simulink model "img_Closedloop"  (R2015b)
settings: Solver=VariableStepAuto  StartTime=0.0  StopTime=600  RelTol=1e-3
values from neighbouring files (symbols this model uses):
  Cp = xlsread(filename)    [Cpfun.m]
undefined symbols (not defined in the file or in its folder): A1, a11, a12, a13, A2, a21, a22, a23, A3, a31, a32, a33, A4, A5, b11, b12, b21, b22, b31, b32, beta_opt, Cr, eta, Jr, lambda, lambda_opt, phi, R, Rho, vf
settings Model: Creator=alino  LastModifiedBy=alino

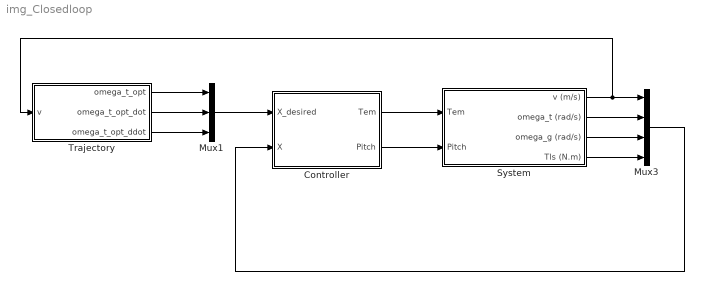
== system img_Closedloop ==
  Controller : Subsystem
  Mux1 : Mux  Inputs=3
  Mux3 : Mux
  System : Subsystem
  Trajectory : Subsystem
  wires:
  Mux3/1 -> Controller/2(X)
  Mux1/1 -> Controller/1(X_desired)
  Trajectory/2(omega_t_opt_dot) -> Mux1/2
  Trajectory/1(omega_t_opt) -> Mux1/1
  Controller/1(Tem) -> System/1(Tem)
  Controller/2(Pitch) -> System/2(Pitch)
  System/3(omega_g (rad/s)) -> Mux3/3
  System/4(Tls (N.m)) -> Mux3/4
  System/2(omega_t (rad/s)) -> Mux3/2
  System/1(v (m/s)) -> Trajectory/1(v), Mux3/1
  Trajectory/3(omega_t_opt_ddot) -> Mux1/3

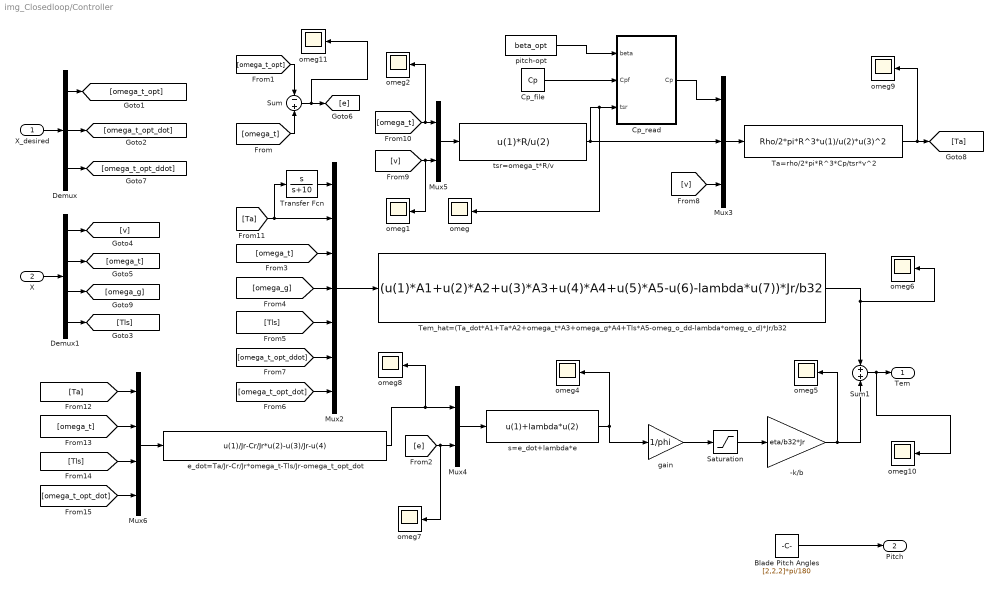
== system img_Closedloop/Controller ==
  X_desired : Inport
  X : Inport  Port=2
  -k/b : Gain  Gain=eta/b32*Jr
  Blade Pitch Angles : Constant  Value=[2,2,2]*pi/180
  Cp_file : Constant  Value=Cp
  Cp_read : MATLAB Function  TreatAsAtomicUnit=on
  Demux : Demux  Outputs=3
  Demux1 : Demux
  Mux2 : Mux  Inputs=7
  Mux3 : Mux  Inputs=3
  Mux4 : Mux  Inputs=2
  Mux5 : Mux  Inputs=2
  Mux6 : Mux
  Saturation : Saturate  UpperLimit=1  LowerLimit=-1
  Sum : Sum  Inputs=-+
  Sum1 : Sum  Inputs=+|+
  Ta=rho/2*pi*R^3*Cp/tsr*v^2 : Fcn  Expr=Rho/2*pi*R^3*u(1)/u(2)*u(3)^2
  Tem_hat=(Ta_dot*A1+Ta*A2+omega_t*A3+omega_g*A4+Tls*A5-omeg_o_dd-lambda*omeg_o_d)*Jr/b32 : Fcn  Expr=(u(1)*A1+u(2)*A2+u(3)*A3+u(4)*A4+u(5)*A5-u(6)-lambda*u(7))*Jr/b32
  Transfer Fcn : TransferFcn  Numerator=[1 0]  Denominator=[1 10]
  e_dot=Ta/Jr-Cr/Jr*omega_t-Tls/Jr-omega_t_opt_dot : Fcn  Expr=u(1)/Jr-Cr/Jr*u(2)-u(3)/Jr-u(4)
  gain : Gain  Gain=1/phi
  omeg{,1..2,4..11} (11 alike) : Scope
  pitch-opt : Constant  Value=beta_opt
  s=e_dot+lambda*e : Fcn  Expr=u(1)+lambda*u(2)
  tsr=omega_t*R/v : Fcn  Expr=u(1)*R/u(2)
  Tem : Outport
  Pitch : Outport  Port=2
  wires:
  X_desired/1 -> Demux/1
  X/1 -> Demux1/1
  Tem_hat=(Ta_dot*A1+Ta*A2+omega_t*A3+omega_g*A4+Tls*A5-omeg_o_dd-lambda*omeg_o_d)*Jr/b32/1 -> Sum1/1, omeg6/1
  -k/b/1 -> Sum1/2, omeg5/1
  Mux2/1 -> Tem_hat=(Ta_dot*A1+Ta*A2+omega_t*A3+omega_g*A4+Tls*A5-omeg_o_dd-lambda*omeg_o_d)*Jr/b32/1
  Mux4/1 -> s=e_dot+lambda*e/1
  [omega_t] -> Mux2/3
  Demux/1 -> [omega_t_opt]
  Demux/2 -> [omega_t_opt_dot]
  Demux1/1 -> [v]
  Demux1/2 -> [omega_t]
  Demux1/3 -> [omega_g]
  Blade Pitch Angles/1 -> Pitch/1
  Demux1/4 -> [Tls]
  Sum/1 -> omeg11/1, [e]
  [omega_t] -> Sum/2
  [omega_t_opt] -> Sum/1
  [e] -> omeg7/1, Mux4/2
  Demux/3 -> [omega_t_opt_ddot]
  [omega_g] -> Mux2/4
  [Tls] -> Mux2/5
  Mux3/1 -> Ta=rho/2*pi*R^3*Cp/tsr*v^2/1
  [v] -> Mux3/3
  Mux5/1 -> tsr=omega_t*R/v/1
  [v] -> omeg1/1, Mux5/2
  [omega_t] -> omeg2/1, Mux5/1
  tsr=omega_t*R/v/1 -> Mux3/2, omeg/1, Cp_read/3(tsr)
  Ta=rho/2*pi*R^3*Cp/tsr*v^2/1 -> omeg9/1, [Ta]
  [Ta] -> Transfer Fcn/1, Mux2/2
  Transfer Fcn/1 -> Mux2/1
  Mux6/1 -> e_dot=Ta/Jr-Cr/Jr*omega_t-Tls/Jr-omega_t_opt_dot/1
  e_dot=Ta/Jr-Cr/Jr*omega_t-Tls/Jr-omega_t_opt_dot/1 -> omeg8/1, Mux4/1
  [Ta] -> Mux6/1
  [omega_t] -> Mux6/2
  [Tls] -> Mux6/3
  [omega_t_opt_dot] -> Mux6/4
  Cp_read/1(Cp) -> Mux3/1
  Cp_file/1 -> Cp_read/2(Cpf)
  pitch-opt/1 -> Cp_read/1(beta)
  Sum1/1 -> omeg10/1, Tem/1
  [omega_t_opt_dot] -> Mux2/7
  [omega_t_opt_ddot] -> Mux2/6
  s=e_dot+lambda*e/1 -> gain/1, omeg4/1
  Saturation/1 -> -k/b/1
  gain/1 -> Saturation/1

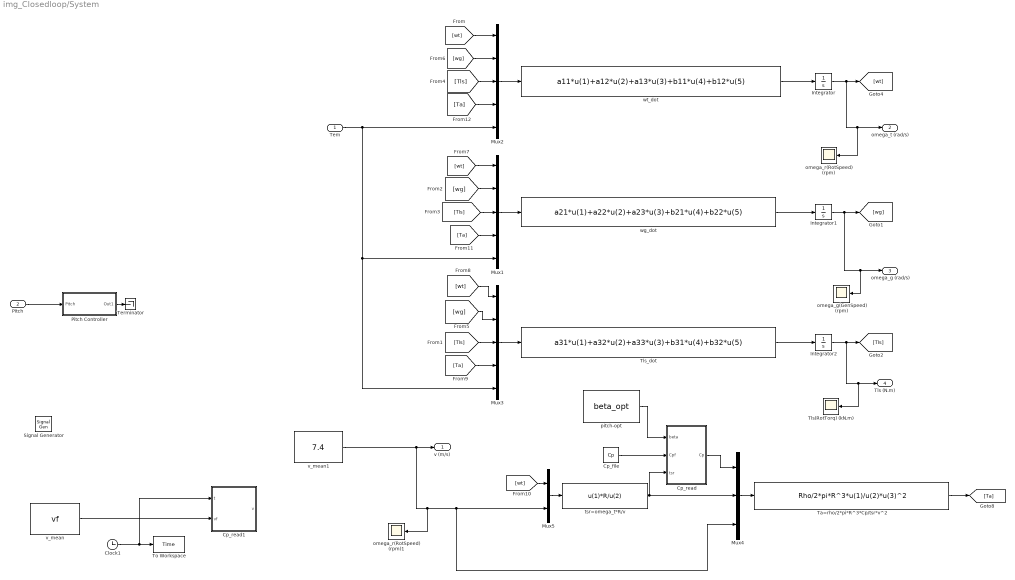
== system img_Closedloop/System ==
  Tem : Inport
  Pitch : Inport  Port=2
  Clock1 : Clock
  Cp_file : Constant  Value=Cp
  Cp_read : MATLAB Function  TreatAsAtomicUnit=on
  Cp_read1 : MATLAB Function  TreatAsAtomicUnit=on
  Integrator : Integrator  InitialCondition=2
  Integrator1 : Integrator  InitialCondition=2
  Integrator2 : Integrator
  Mux1 : Mux  Inputs=5
  Mux2 : Mux  Inputs=5
  Mux3 : Mux  Inputs=5
  Mux4 : Mux  Inputs=3
  Mux5 : Mux  Inputs=2
  Pitch Controller : Subsystem
  Signal Generator : SignalGenerator  WaveForm=random  Units=rad/sec
  Ta=rho/2*pi*R^3*Cp/tsr*v^2 : Fcn  Expr=Rho/2*pi*R^3*u(1)/u(2)*u(3)^2
  Terminator : Terminator
  Tls(RotTorq) (kN.m) : Scope
  Tls_dot : Fcn  Expr=a31*u(1)+a32*u(2)+a33*u(3)+b31*u(4)+b32*u(5)
  To Workspace : ToWorkspace  VariableName=Time  SampleTime=-1
  omega_g(GenSpeed) (rpm) : Scope
  omega_r(RotSpeed) (rpm) : Scope
  omega_r(RotSpeed) (rpm)1 : Scope
  pitch-opt : Constant  Value=beta_opt
  tsr=omega_t*R/v : Fcn  Expr=u(1)*R/u(2)
  v_mean : Constant  Value=vf
  v_mean1 : Constant  Value=7.4
  wg_dot : Fcn  Expr=a21*u(1)+a22*u(2)+a23*u(3)+b21*u(4)+b22*u(5)
  wt_dot : Fcn  Expr=a11*u(1)+a12*u(2)+a13*u(3)+b11*u(4)+b12*u(5)
  v (m/s) : Outport
  omega_t (rad/s) : Outport  Port=2
  omega_g (rad/s) : Outport  Port=3
  Tls (N.m) : Outport  Port=4
  wires:
  Clock1/1 -> Cp_read1/1(t), To Workspace/1
  Integrator/1 -> omega_t (rad/s)/1, omega_r(RotSpeed) (rpm)/1, [wt]
  Integrator1/1 -> omega_g(GenSpeed) (rpm)/1, omega_g (rad/s)/1, [wg]
  Integrator2/1 -> Tls(RotTorq) (kN.m)/1, Tls (N.m)/1, [Tls]
  Pitch/1 -> Pitch Controller/1(Pitch)
  Mux2/1 -> wt_dot/1
  Mux1/1 -> wg_dot/1
  Mux3/1 -> Tls_dot/1
  wt_dot/1 -> Integrator/1
  [wt] -> Mux2/1
  wg_dot/1 -> Integrator1/1
  Tls_dot/1 -> Integrator2/1
  [wt] -> Mux3/1
  [wg] -> Mux1/2
  [Tls] -> Mux3/3
  [Tls] -> Mux1/3
  [Tls] -> Mux2/3
  [wg] -> Mux3/2
  [wg] -> Mux2/2
  [wt] -> Mux1/1
  Tem/1 -> Mux3/5, Mux1/5, Mux2/5
  Pitch Controller/1(Out1) -> Terminator/1
  Mux4/1 -> Ta=rho/2*pi*R^3*Cp/tsr*v^2/1
  v_mean1/1 -> omega_r(RotSpeed) (rpm)1/1, Mux4/3, Mux5/2, v (m/s)/1
  Mux5/1 -> tsr=omega_t*R/v/1
  [wt] -> Mux5/1
  tsr=omega_t*R/v/1 -> Mux4/2, Cp_read/3(tsr)
  Ta=rho/2*pi*R^3*Cp/tsr*v^2/1 -> [Ta]
  Cp_read/1(Cp) -> Mux4/1
  Cp_file/1 -> Cp_read/2(Cpf)
  pitch-opt/1 -> Cp_read/1(beta)
  [Ta] -> Mux3/4
  [Ta] -> Mux1/4
  [Ta] -> Mux2/4
  v_mean/1 -> Cp_read1/2(vf)

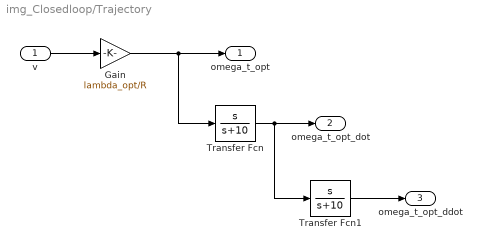
== system img_Closedloop/Trajectory ==
  v : Inport
  Gain : Gain  Gain=lambda_opt/R
  Transfer Fcn : TransferFcn  Numerator=[1 0]  Denominator=[1 10]
  Transfer Fcn1 : TransferFcn  Numerator=[1 0]  Denominator=[1 10]
  omega_t_opt : Outport
  omega_t_opt_dot : Outport  Port=2
  omega_t_opt_ddot : Outport  Port=3
  wires:
  Transfer Fcn/1 -> Transfer Fcn1/1, omega_t_opt_dot/1
  v/1 -> Gain/1
  Gain/1 -> Transfer Fcn/1, omega_t_opt/1
  Transfer Fcn1/1 -> omega_t_opt_ddot/1

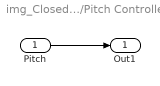
== system img_Closedloop/System/Pitch Controller ==
  Pitch : Inport
  Out1 : Outport
  wires:
  Pitch/1 -> Out1/1

== matlab function img_Closedloop/Controller/Cp_read ==
  data: beta input; Cpf input; Cp output; tsr input
function Cp = fcn(beta,Cpf,tsr)

    if (tsr>19 || beta>90) 
        Cp=0;
    else
    beta1=floor(beta)+1;
    tsr1=floor(tsr*10);
    beta2=beta1+1;
    tsr2=tsr1+1;
    betap=beta-floor(beta);
    tsrp=tsr*10-floor(tsr*10);
    Cp1=Cpf(beta1,tsr1)+betap*(Cpf(beta2,tsr1)-Cpf(beta1,tsr1));
    Cp2=Cpf(beta1,tsr2)+betap*(Cpf(beta2,tsr2)-Cpf(beta1,tsr2));
    Cp=tsrp*(Cp2-Cp1)+Cp1;
    end
end

== matlab function img_Closedloop/System/Cp_read1 ==
  data: t input; v output; vf input
function v = fcn(t,vf)
    v=vf(floor(2*t)+1);
end

== matlab function img_Closedloop/System/Cp_read ==
  data: beta input; Cpf input; Cp output; tsr input
function Cp = fcn(beta,Cpf,tsr)

    if (tsr>19) || (beta>90) || (tsr<1) 
        Cp=0;
    else
    beta1=floor(beta)+1;
    tsr1=floor(tsr*10);
    beta2=beta1+1;
    tsr2=tsr1+1;
    betap=beta-floor(beta);
    tsrp=tsr*10-floor(tsr*10);
    Cp1=Cpf(beta1,tsr1)+betap*(Cpf(beta2,tsr1)-Cpf(beta1,tsr1));
    Cp2=Cpf(beta1,tsr2)+betap*(Cpf(beta2,tsr2)-Cpf(beta1,tsr2));
    Cp=tsrp*(Cp2-Cp1)+Cp1;
    end
end
